simulink model "ECE551_poleplacement_ex_2017"  (R2017b)
settings: Solver=VariableStepAuto  StartTime=0.0  StopTime=10.0  RelTol=1e-3
values from neighbouring files (symbols this model uses):
  a = 0.0043    [ECE531HW1.m]    (also in ECE551_ex2.m = [1 2]; ECE551_ex3.m = [1,0;0,-3]; ECE551_ex4.m = [0,1;0,0]; ECE580_HW4.m = 1*exp(j*120/pol))
  b = {(1), (2)}    [ECE551_ex2.m]    (also in ECE551_ex3.m = [1;1]; ECE551_ex4.m = [0;1]; ECE580_HW4.m = linspace(0,1) * (Zlt/ZTR))
  c = 385    [ECE531HW1.m]    (also in ECE551_ex2.m = {{1}, {'hello'}}; ECE551_ex4.m = [1,0])
  cx = eye(size(a))    [ECE551_ex4.m]
  dx = zeros(size(b))    [ECE551_ex4.m]
  k = place(A,Bd,P)    [ECE551_Project_part2.m]    (also in ECE551_ex4.m = acker(a,b,p); ECE_580_HW2.m = [1:Nsc])
settings Model: Creator=clarke6  LastModifiedBy=clarke6

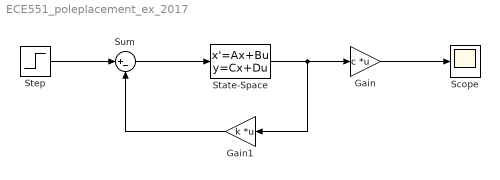
== system ECE551_poleplacement_ex_2017 ==
  Gain : Gain  Gain=c  Multiplication=Matrix(K*u)
  Gain1 : Gain  Gain=k  Multiplication=Matrix(K*u)
  Scope : Scope
  State-Space : StateSpace  A=a  B=b  C=cx  D=dx  InitialCondition=0
  Step : Step  SampleTime=0
  Sum : Sum  Inputs=|+-
  wires:
  Step/1 -> Sum/1
  Sum/1 -> State-Space/1
  State-Space/1 -> Gain1/1, Gain/1
  Gain/1 -> Scope/1
  Gain1/1 -> Sum/2
